simulink model "proxy_linux"  (R2017b)
settings: Solver=ode3  StartTime=0.0  StopTime=inf  FixedStep=0.01  RelTol=1e-3  EnableMultiTasking=on
model workspace (MAT data in the model file):
  SL_ROS_VariableLengthArrays_MaxSizes.CommonInfo.ArrayTruncateAction = 'EmitWarning'
  SL_ROS_VariableLengthArrays_MaxSizes.MsgTypeMap = containers.Map
  SL_ROS_VariableLengthArrays_MaxSizes.MsgTypeMap.serialization.keys = {'std_msgs/Float32MultiArray'}
  SL_ROS_VariableLengthArrays_MaxSizes.MsgTypeMap.serialization.values{1}.PropertyName = 'Data'
  SL_ROS_VariableLengthArrays_MaxSizes.MsgTypeMap.serialization.values{1}.DataType = 'single'
  SL_ROS_VariableLengthArrays_MaxSizes.MsgTypeMap.serialization.values{1}.MaxLength = 2
  SL_ROS_VariableLengthArrays_MaxSizes.MsgTypeMap.serialization.uniformity = 0
  SL_ROS_VariableLengthArrays_MaxSizes.MsgTypeMap.serialization.keyType = 'char'
  SL_ROS_VariableLengthArrays_MaxSizes.MsgTypeMap.serialization.valueType = 'any'
undefined symbols (not defined in the file or in its folder): ampliFactor, ampliFactorDistal, ampliFactorMiddle, filt
libraries: robotlib x11, simulink_extras x11, simulink x8, etargetslib x4, dspnetwork x4
(part 1 of 6)
settings Model: Creator=Centauro  LastModifiedBy=Centauro
settings DataIOCC: LimitDataPoints=on  SaveFormat=Array
settings OptimizationCC: PassReuseOutputArgsThreshold=0  MaxStackSize=64
settings DebuggingCC: ParameterTunabilityLossMsg=error  SFUnexpectedBacktrackingDiag=warning  SFNoUnconditionalDefaultTransitionDiag=warning  SFExecutionAtInitializationDiag=none
settings HardwareCC: ProdBitPerPointer=32  ProdBitPerSizeT=32  ProdBitPerPtrDiffT=32  ProdLargestAtomicFloat=None  ProdIntDivRoundTo=Undefined  ProdEndianess=Unspecified  ProdWordSize=32  ProdHWDeviceType=Generic->Unspecified (assume 32-bit Generic)  UseEmbeddedCoderFeatures=off
settings ModelReferenceCC: PropagateSignalLabelsOutOfModel=off
settings SFSimCC: MATLABDynamicMemAlloc=off
settings RTWCC: SystemTargetFile=ert.tlc  HardwareBoard=Robot Operating System (ROS)  TemplateMakefile=ert_default_tmf  GenerateReport=on  Toolchain=Catkin  LaunchReport=on  TargetLang=C++
settings CodeAppCC: ForceParamTrailComments=on  OperatorAnnotations=on
settings ERTTargetCC: ERTCustomFileBanners=off  SupportContinuousTime=on  SupportNonInlinedSFcns=on  RemoveResetFunc=off  ModelStepFunctionPrototypeControlCompliant=off
settings ConfigComp: CovMetricSettings=dw  CovHtmlReporting=on  CovSaveCumulativeToWorkspaceVar=on  CovSaveSingleToWorkspaceVar=on  CovExternalEMLEnable=off

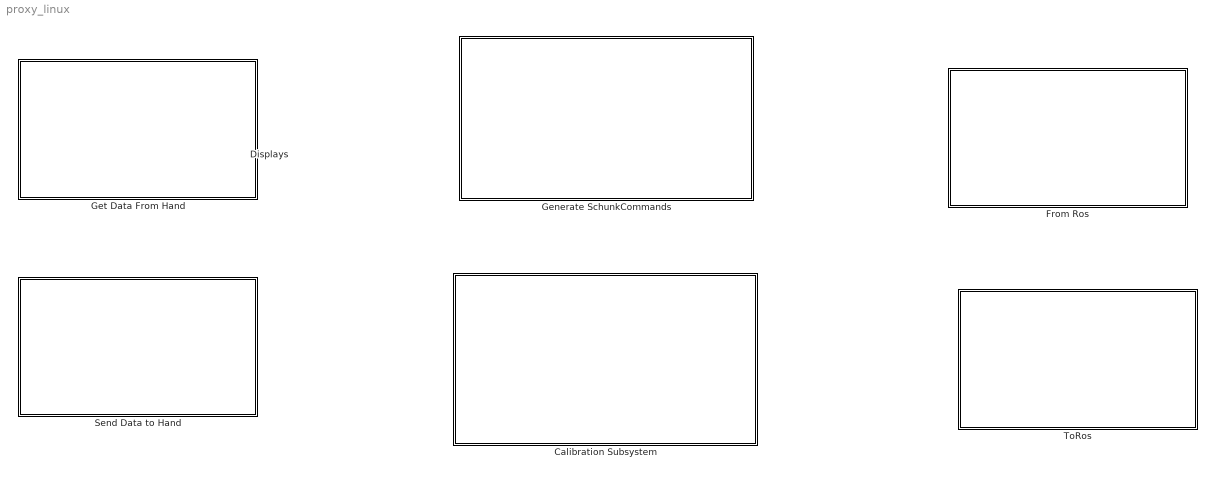
== system proxy_linux ==
  Calibration Subsystem : Subsystem
  "Displays " : Subsystem
  From Ros : Subsystem
  "Generate SchunkCommands " : Subsystem
  Get Data From Hand : Subsystem
  Send Data to Hand : Subsystem
  ToRos : Subsystem

== system proxy_linux/Calibration Subsystem ==
  Bus Selector : BusSelector  OutputSignals=Data
  Chart : Stateflow chart  Commented=on  TreatAsAtomicUnit=on
  Constant : Constant  Value=true  OutDataTypeStr=boolean
  Display : Display
  From1 : From  Commented=on  GotoTag=Index_Precalibration  TagVisibility=global
  From2 : From  Commented=on  GotoTag=Middle_Precalibration
  Goto1 : Goto  Commented=on  GotoTag=CalibrationSignal  TagVisibility=global
  Goto2 : Goto  Commented=on  GotoTag=IndexCalibrationOffset  TagVisibility=global
  Goto3 : Goto  Commented=on  GotoTag=MiddleCalibrationOffset  TagVisibility=global
  Logical Operator : Logic  Operator=NOT  AllPortsSameDT=off  OutDataTypeStr=boolean
  Manual Switch : ManualSwitch  CurrentSetting=0
  Memory : Memory  Commented=on
  Memory1 : Memory  Commented=on
  Memory2 : Memory  Commented=on
  Subscribe1 : robotlib/Subscribe  SourceLibraryInfo=This block requires Robotics System Toolbox  topicSource=Select from ROS network  topic=/left_hand/button_1  messageType=std_msgs/Bool  sampleTime=0.01  messageQueueLength=1
      settings: SourceProductBaseCode=RO
  Terminator : Terminator
  tag scope: CalibrationSignal=global
  wires:
  Subscribe1/1 -> Terminator/1
  Subscribe1/2 -> Bus Selector/1
  From1/1 -> Chart/1(IndexPrescaler)
  From2/1 -> Chart/2(MiddlePrescaler)
  Chart/2(MiddleOffset) -> Memory1/1
  Chart/1(IndexOffset) -> Memory/1
  Chart/3(CalibrationDone) -> Memory2/1
  Memory/1 -> Goto2/1
  Memory1/1 -> Goto3/1
  Memory2/1 -> Goto1/1
  Logical Operator/1 -> [CalibrationSignal], Chart/3(Calibration), Display/1
  Manual Switch/1 -> Logical Operator/1
  Bus Selector/1 -> Manual Switch/2  "<Data>"
  Constant/1 -> Manual Switch/1

== system proxy_linux/Displays  ==
  Display{,1..3} (4 alike) : Display
  wires:
  [Forces] -> Display1/1
  [RotativePot] -> Display3/1
  [Header] -> Display/1
  [MotorsPot] -> Display2/1

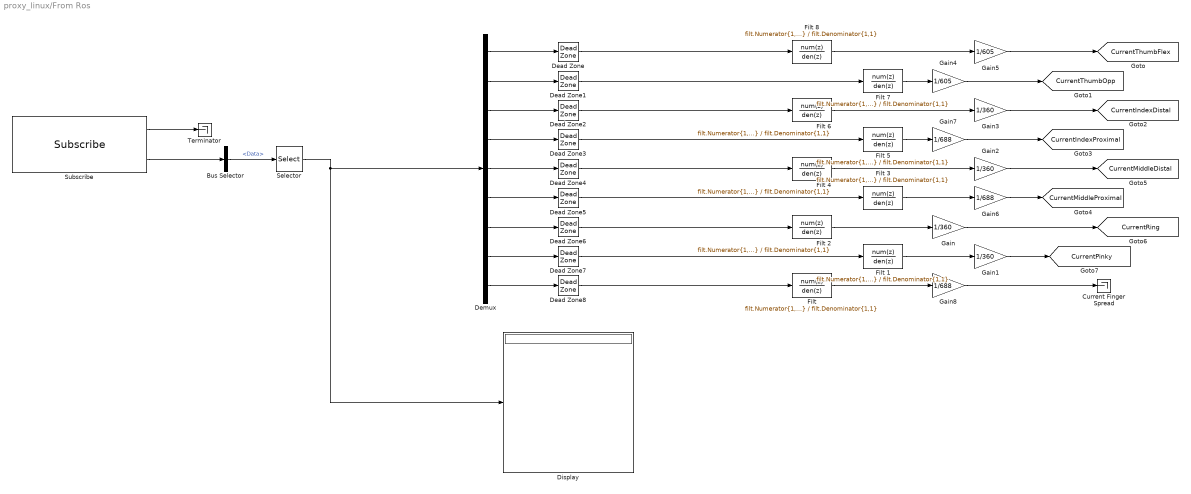
== system proxy_linux/From Ros ==
  Bus Selector : BusSelector  OutputSignals=Data
  Current Finger Spread : Terminator
  Dead Zone{,1..8} (9 alike) : DeadZone  LowerValue=-30  UpperValue=30  SaturateOnIntegerOverflow=on
  Demux : Demux  Outputs=9
  Display : Display
  Filt {,1..8} (9 alike) : DiscreteTransferFcn  Numerator=filt.Numerator{1,1}  Denominator=filt.Denominator{1,1}  SampleTime=0.01
  Gain{,1..3} (4 alike) : Gain  Gain=1/360
  Gain4 : Gain  Gain=1/605
  Gain5 : Gain  Gain=1/605
  Gain6 : Gain  Gain=1/688
  Gain7 : Gain  Gain=1/688
  Gain8 : Gain  Gain=1/688
  Selector : Selector  IndexOptions=Index vector (dialog)  Indices=[1 2 3 4 5 6 7 8 9]  OutputSizes=1
  Subscribe : robotlib/Subscribe  SourceLibraryInfo=This block requires Robotics System Toolbox  topicSource=Select from ROS network  topic=/svh_controller/channel_currents  messageType=std_msgs/Float64MultiArray  sampleTime=0.01  messageQueueLength=1
      settings: SourceProductBaseCode=RO
  Terminator : Terminator
  tag scope: CurrentIndexDistal=global, CurrentIndexProximal=global, CurrentMiddleDistal=global, CurrentMiddleProximal=global, CurrentPinky=global, CurrentRing=global, CurrentThumbFlex=global, CurrentThumbOpp=global
  wires:
  Subscribe/1 -> Terminator/1
  Subscribe/2 -> Bus Selector/1
  Bus Selector/1 -> Selector/1  "<Data>"
  Selector/1 -> Demux/1, Display/1
  Demux/1 -> Dead Zone/1
  Demux/2 -> Dead Zone1/1
  Demux/3 -> Dead Zone2/1
  Demux/4 -> Dead Zone3/1
  Demux/6 -> Dead Zone5/1
  Demux/5 -> Dead Zone4/1
  Demux/7 -> Dead Zone6/1
  Demux/8 -> Dead Zone7/1
  Demux/9 -> Dead Zone8/1
  "Filt "/1 -> Gain8/1
  Filt 1/1 -> Gain1/1
  Filt 2/1 -> Gain/1
  Filt 4/1 -> Gain2/1
  Filt 5/1 -> Gain7/1
  Filt 6/1 -> Gain3/1
  Filt 7/1 -> Gain4/1
  Filt 8/1 -> Gain5/1
  Gain1/1 -> [CurrentPinky]
  Gain/1 -> [CurrentRing]
  Filt 3/1 -> Gain6/1
  Gain2/1 -> [CurrentMiddleDistal]
  Gain3/1 -> [CurrentIndexDistal]
  Gain5/1 -> [CurrentThumbFlex]
  Gain4/1 -> [CurrentThumbOpp]
  Gain7/1 -> [CurrentIndexProximal]
  Gain6/1 -> [CurrentMiddleProximal]
  Gain8/1 -> Current Finger Spread/1
  Dead Zone/1 -> Filt 8/1
  Dead Zone1/1 -> Filt 7/1
  Dead Zone2/1 -> Filt 6/1
  Dead Zone3/1 -> Filt 5/1
  Dead Zone4/1 -> Filt 4/1
  Dead Zone5/1 -> Filt 3/1
  Dead Zone6/1 -> Filt 2/1
  Dead Zone7/1 -> Filt 1/1
  Dead Zone8/1 -> "Filt "/1

== system proxy_linux/Generate SchunkCommands  ==
  Finger Spread : Subsystem
  Index : Subsystem
  Index Finger : Subsystem  Commented=on
  Middle Finger : Subsystem
  Pinky : Subsystem
  "Ring " : Subsystem
  Thumb : Subsystem

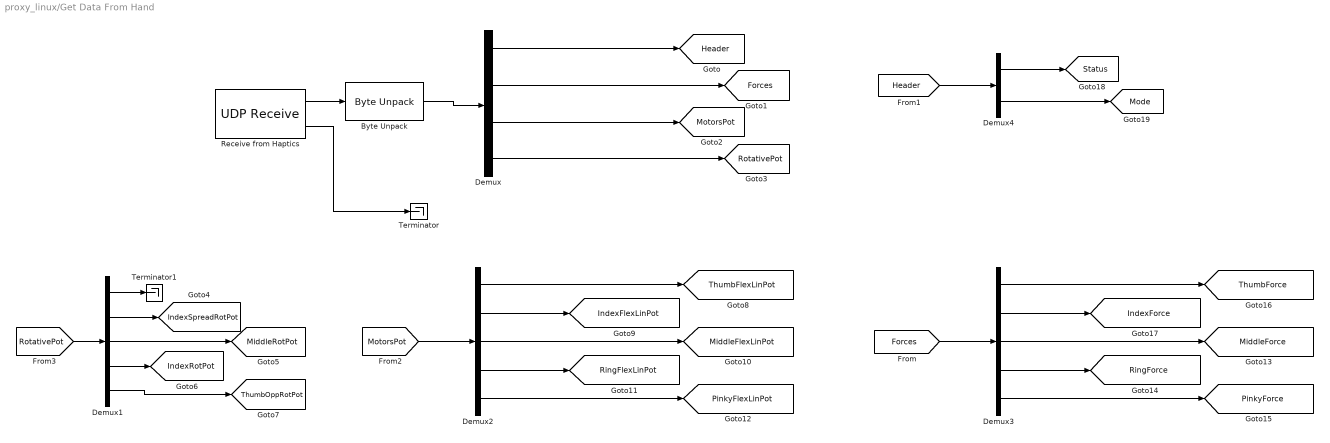
== system proxy_linux/Get Data From Hand ==
  Byte Unpack : etargetslib/Byte Unpack  dimensions={[17]}  datatypes={'single'}  byteAlign=1
  Demux : Demux  Outputs=[2, 5, 5, 5]
  Demux1 : Demux  Outputs=5
  Demux2 : Demux  Outputs=5
  Demux3 : Demux  Outputs=5
  Demux4 : Demux  Outputs=2
  Receive from Haptics : dspnetwork/UDP Receive  localURL='0.0.0.0'  localPort=15001  remoteURL=RightHandAddress  remotePort=-1  recvBufferSize=17*4  dims=17*4  signalDatatype=uint8  isVarSize=off  showBlockingTime=on  blockingTime=inf  sampletime=0.01  blockPlatform=HOST
      settings: SourceProductName=DSP System Toolbox  SourceProductBaseCode=DS
  Terminator : Terminator
  Terminator1 : Terminator
  tag scope: Forces=global, Header=global, IndexFlexLinPot=global, IndexForce=global, IndexRotPot=global, IndexSpreadRotPot=global, MiddleFlexLinPot=global, MiddleForce=global, MiddleRotPot=global, Mode=global, MotorsPot=global, PinkyFlexLinPot=global, PinkyForce=global, RingFlexLinPot=global, RingForce=global, RotativePot=global, Status=global, ThumbFlexLinPot=global, ThumbForce=global, ThumbOppRotPot=global
  wires:
  Demux/3 -> [MotorsPot]
  Demux/1 -> [Header]
  Demux/4 -> [RotativePot]
  Demux/2 -> [Forces]
  Receive from Haptics/2 -> Terminator/1
  [RotativePot] -> Demux1/1
  Demux1/2 -> [IndexSpreadRotPot]
  Demux1/3 -> [MiddleRotPot]
  Demux1/4 -> [IndexRotPot]
  Demux1/5 -> [ThumbOppRotPot]
  Demux1/1 -> Terminator1/1
  Demux2/1 -> [ThumbFlexLinPot]
  Demux2/2 -> [IndexFlexLinPot]
  [MotorsPot] -> Demux2/1
  Demux2/3 -> [MiddleFlexLinPot]
  Demux2/4 -> [RingFlexLinPot]
  Demux2/5 -> [PinkyFlexLinPot]
  Demux3/1 -> [ThumbForce]
  Demux3/2 -> [IndexForce]
  [Forces] -> Demux3/1
  Demux3/3 -> [MiddleForce]
  Demux3/4 -> [RingForce]
  Demux3/5 -> [PinkyForce]
  [Header] -> Demux4/1
  Demux4/1 -> [Status]
  Demux4/2 -> [Mode]
  Byte Unpack/1 -> Demux/1
  Receive from Haptics/1 -> Byte Unpack/1

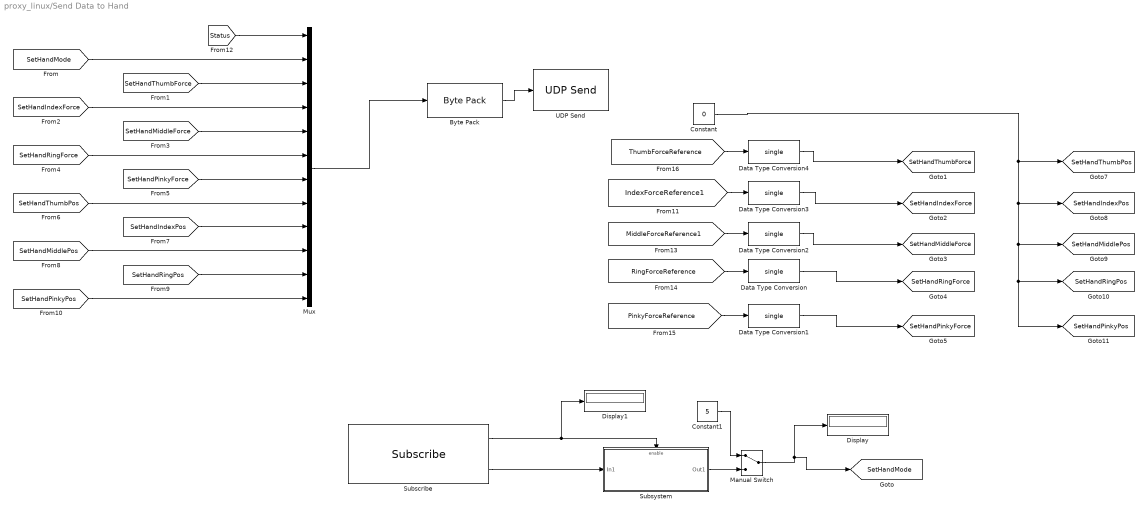
== system proxy_linux/Send Data to Hand ==
  Byte Pack : etargetslib/Byte Pack  datatypes={'single'}  byteAlign=1
  Constant : Constant  Value=0  OutDataTypeStr=single
  Constant1 : Constant  Value=5  OutDataTypeStr=single
  Data Type Conversion{,1..4} (5 alike) : DataTypeConversion  OutDataTypeStr=single
  Display : Display
  Display1 : Display
  Manual Switch : ManualSwitch
  Mux : Mux  Inputs=12
  Subscribe : robotlib/Subscribe  SourceLibraryInfo=This block requires Robotics System Toolbox  topicSource=Specify your own  topic=/manual_commands/rh_mode  messageType=std_msgs/Float64  sampleTime=-1  messageQueueLength=1
      settings: SourceProductBaseCode=RO
  Subsystem : Subsystem
  UDP Send : dspnetwork/UDP Send  remoteURL=RightHandAddress  remotePort=12000  localURL='0.0.0.0'  localPortSource=Automatically determine  localPort=-1  sampletime=-1  blockPlatform=HOST  separateLengthPort=0
      settings: SourceProductName=DSP System Toolbox  SourceProductBaseCode=DS
  tag scope: SetHandIndexForce=global, SetHandIndexPos=global, SetHandMiddleForce=global, SetHandMiddlePos=global, SetHandMode=global, SetHandPinkyForce=global, SetHandPinkyPos=global, SetHandRingForce=global, SetHandRingPos=global, SetHandThumbForce=global, SetHandThumbPos=global
  wires:
  Byte Pack/1 -> UDP Send/1
  [SetHandMode] -> Mux/2
  [SetHandThumbForce] -> Mux/3
  [SetHandIndexForce] -> Mux/4
  [SetHandRingForce] -> Mux/6
  [SetHandMiddleForce] -> Mux/5
  [SetHandPinkyForce] -> Mux/7
  [SetHandThumbPos] -> Mux/8
  [SetHandIndexPos] -> Mux/9
  [SetHandMiddlePos] -> Mux/10
  [SetHandRingPos] -> Mux/11
  [SetHandPinkyPos] -> Mux/12
  [Status] -> Mux/1
  [ThumbForceReference] -> Data Type Conversion4/1
  [RingForceReference] -> Data Type Conversion/1
  [PinkyForceReference] -> Data Type Conversion1/1
  [MiddleForceReference1] -> Data Type Conversion2/1
  [IndexForceReference1] -> Data Type Conversion3/1
  Constant/1 -> [SetHandThumbPos], [SetHandIndexPos], [SetHandMiddlePos], [SetHandRingPos], [SetHandPinkyPos]
  Mux/1 -> Byte Pack/1
  Subscribe/2 -> Subsystem/1(In1)
  Subscribe/1 -> Display1/1, Subsystem/Enable
  Data Type Conversion/1 -> [SetHandRingForce]
  Data Type Conversion1/1 -> [SetHandPinkyForce]
  Data Type Conversion2/1 -> [SetHandMiddleForce]
  Data Type Conversion3/1 -> [SetHandIndexForce]
  Data Type Conversion4/1 -> [SetHandThumbForce]
  Subsystem/1(Out1) -> Manual Switch/2
  Constant1/1 -> Manual Switch/1
  Manual Switch/1 -> [SetHandMode], Display/1

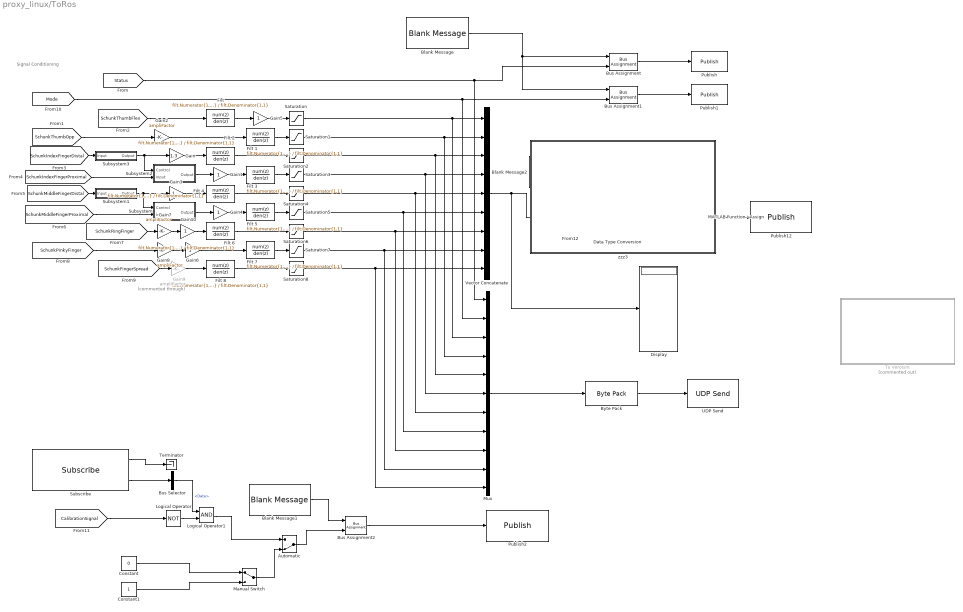
== system proxy_linux/ToRos ==
  note: Signal Conditioning
  "Automatic " : ManualSwitch  CurrentSetting=0
  Blank Message : robotlib/Blank Message  SourceLibraryInfo=This block requires Robotics System Toolbox  messageType=std_msgs/Float32  SampleTime=0.01
      settings: SourceProductBaseCode=RO
  Blank Message1 : robotlib/Blank Message  SourceLibraryInfo=This block requires Robotics System Toolbox  messageType=std_msgs/Bool  SampleTime=inf
      settings: SourceProductBaseCode=RO
  Blank Message2 : robotlib/Blank Message  SourceLibraryInfo=This block requires Robotics System Toolbox  messageType=sensor_msgs/JointState  SampleTime=inf
      settings: SourceProductBaseCode=RO
  Bus Assignment : BusAssignment  AssignedSignals=Data
  Bus Assignment1 : BusAssignment  AssignedSignals=Data
  Bus Assignment2 : BusAssignment  AssignedSignals=Data
  Bus Selector : BusSelector  OutputSignals=Data
  Byte Pack : etargetslib/Byte Pack  datatypes={'single'}  byteAlign=1
  Constant : Constant  Value=0  OutDataTypeStr=boolean
  Constant1 : Constant  OutDataTypeStr=boolean
  Data Type Conversion : DataTypeConversion  OutDataTypeStr=uint32
  Display : Display
  Filt {,1..8} (9 alike) : DiscreteTransferFcn  Numerator=filt.Numerator{1,1}  Denominator=filt.Denominator{1,1}  SampleTime=0.01
  Gain : Gain  Gain=1.3
  Gain{1,3..6,10} (6 alike) : Gain
  Gain2 : Gain  Gain=ampliFactor
  Gain7 : Gain  Gain=ampliFactor
  Gain8 : Gain  Gain=ampliFactor
  Gain9 : Gain  Commented=through  Gain=ampliFactor
  Logical Operator : Logic  Operator=NOT  AllPortsSameDT=off  OutDataTypeStr=boolean
  Logical Operator1 : Logic  AllPortsSameDT=off  OutDataTypeStr=boolean
  MATLAB Function - Assign : MATLAB Function  TreatAsAtomicUnit=on
  Manual Switch : ManualSwitch
  Mux : Mux  Inputs=11
  Publish : robotlib/Publish  SourceLibraryInfo=This block requires Robotics System Toolbox  topicSource=Specify your own  topic=/MatlabStatus  messageType=std_msgs/Float32  messageQueueLength=1
      settings: SourceProductBaseCode=RO
  Publish1 : robotlib/Publish  SourceLibraryInfo=This block requires Robotics System Toolbox  topicSource=Specify your own  topic=/MatlabMode  messageType=std_msgs/Float32  messageQueueLength=1
      settings: SourceProductBaseCode=RO
  Publish12 : robotlib/Publish  SourceLibraryInfo=This block requires Robotics System Toolbox  topicSource=Specify your own  topic=/scan  messageType=sensor_msgs/JointState  messageQueueLength=1
      settings: SourceProductBaseCode=RO
  Publish2 : robotlib/Publish  SourceLibraryInfo=This block requires Robotics System Toolbox  topicSource=Specify your own  topic=/trigger_exo_hand  messageType=std_msgs/Bool  messageQueueLength=1
      settings: SourceProductBaseCode=RO
  Saturation : Saturate  UpperLimit=0.97  LowerLimit=0
  Saturation1 : Saturate  UpperLimit=0.99  LowerLimit=0
  Saturation2 : Saturate  UpperLimit=1.33  LowerLimit=0
  Saturation3 : Saturate  UpperLimit=0.80  LowerLimit=0
  Saturation4 : Saturate  UpperLimit=1.33  LowerLimit=0
  Saturation5 : Saturate  UpperLimit=0.80  LowerLimit=0
  Saturation6 : Saturate  UpperLimit=0.98  LowerLimit=0
  Saturation7 : Saturate  UpperLimit=0.98  LowerLimit=0
  Saturation8 : Saturate  UpperLimit=0.30  LowerLimit=0.05
  Subscribe : robotlib/Subscribe  SourceLibraryInfo=This block requires Robotics System Toolbox  topicSource=Specify your own  topic=/manual_commands/start  messageType=std_msgs/Bool  sampleTime=0.01  messageQueueLength=1
      settings: SourceProductBaseCode=RO
  Subsystem : Subsystem
  Subsystem1 : Subsystem
  Subsystem2 : Subsystem
  Subsystem3 : Subsystem
  Terminator : Terminator
  To Verosim : Subsystem  Commented=on
  UDP Send : dspnetwork/UDP Send  remoteURL=Verosim  remotePort=15000  localURL='0.0.0.0'  localPortSource=Automatically determine  localPort=-1  sampletime=-1  blockPlatform=HOST  separateLengthPort=0
      settings: SourceProductName=DSP System Toolbox  SourceProductBaseCode=DS
  Vector Concatenate : Concatenate  NumInputs=9
  zzz3 : Subsystem  TreatAsAtomicUnit=on
      settings: OpenFcn=% no-op
      mask Display: disp('')
  wires:
  Bus Assignment/1 -> Publish/1
  Blank Message/1 -> Bus Assignment1/1, Bus Assignment/1
  Bus Assignment1/1 -> Publish1/1
  MATLAB Function - Assign/1(msg) -> Publish12/1
  "Filt "/1 -> Gain5/1
  Filt 5/1 -> Saturation5/1
  Filt 6/1 -> Saturation6/1
  Filt 3/1 -> Saturation3/1
  Filt 2/1 -> Saturation2/1
  Filt 4/1 -> Saturation4/1
  Filt 8/1 -> Saturation8/1
  Filt 1/1 -> Saturation1/1
  Filt 7/1 -> Saturation7/1
  [SchunkThumbFlex] -> "Filt "/1
  Gain7/1 -> Gain10/1
  [SchunkFingerSpread] -> Gain9/1
  Gain2/1 -> Filt 1/1
  [SchunkPinkyFinger] -> Gain8/1
  [SchunkThumbOpp] -> Gain2/1
  [SchunkRingFinger] -> Gain7/1
  Gain8/1 -> Gain6/1
  Gain9/1 -> Filt 8/1
  Subsystem3/1(Output) -> Subsystem2/1(Control), Gain/1
  [SchunkMiddleFingerProximal] -> Subsystem/2(Input)
  Bus Assignment2/1 -> Publish2/1
  [CalibrationSignal] -> Logical Operator/1
  Manual Switch/1 -> "Automatic "/2
  Blank Message1/1 -> Bus Assignment2/1
  Constant/1 -> Manual Switch/1
  "Automatic "/1 -> Bus Assignment2/2
  Constant1/1 -> Manual Switch/2
  Vector Concatenate/1 -> Display/1, MATLAB Function - Assign/2(u)
  Subsystem/1("Output ") -> Gain4/1
  [SchunkMiddleFingerDistal] -> Subsystem1/1(Input)
  Subsystem1/1(Output) -> Subsystem/1(Control), Gain3/1
  Saturation/1 -> Mux/3, Vector Concatenate/1
  Saturation1/1 -> Mux/4, Vector Concatenate/2
  Byte Pack/1 -> UDP Send/1
  [Mode] -> Bus Assignment1/2, Mux/2
  [Status] -> Bus Assignment/2, Mux/1
  Saturation5/1 -> Mux/8, Vector Concatenate/6
  Saturation8/1 -> Mux/11, Vector Concatenate/9
  Saturation2/1 -> Mux/5, Vector Concatenate/3
  Saturation3/1 -> Mux/6, Vector Concatenate/4
  Saturation6/1 -> Mux/9, Vector Concatenate/7
  Saturation7/1 -> Mux/10, Vector Concatenate/8
  Saturation4/1 -> Mux/7, Vector Concatenate/5
  Mux/1 -> Byte Pack/1
  Subsystem2/1("Output ") -> Gain1/1
  [SchunkIndexFingerProximal] -> Subsystem2/2(Input)
  [SchunkIndexFingerDistal] -> Subsystem3/1(Input)
  Logical Operator/1 -> Logical Operator1/2
  Logical Operator1/1 -> "Automatic "/1
  Bus Selector/1 -> Logical Operator1/1  "<Data>"
  Subscribe/1 -> Terminator/1
  Subscribe/2 -> Bus Selector/1
  Gain/1 -> Filt 2/1
  Blank Message2/1 -> MATLAB Function - Assign/1(blankMessage)
  Data Type Conversion/1 -> MATLAB Function - Assign/3(timeStamp)
  [Status] -> Data Type Conversion/1
  Gain1/1 -> Filt 3/1
  Gain3/1 -> Filt 4/1
  Gain4/1 -> Filt 5/1
  Gain5/1 -> Saturation/1
  Gain6/1 -> Filt 7/1
  Gain10/1 -> Filt 6/1

== system proxy_linux/Generate SchunkCommands /Finger Spread ==
  Constant : Constant  Value=0.30  OutDataTypeStr=single
  Constant1 : Constant  Value=0.10  OutDataTypeStr=single
  Display : Display
  MATLAB Function : MATLAB Function  TreatAsAtomicUnit=on
  Manual Switch : ManualSwitch
  Mux : Mux  Inputs=2
  Sum : Sum  Inputs=|++
  calibration1 : Subsystem
  tag scope: SchunkFingerSpread=global
  wires:
  [IndexSpreadRotPot] -> calibration1/1(In1), MATLAB Function/1(u)
  Constant/1 -> Manual Switch/2
  MATLAB Function/1(y) -> Manual Switch/1
  calibration1/1(Out1) -> Mux/2, MATLAB Function/2(calib)
  Mux/1 -> Display/1
  Manual Switch/1 -> Sum/1
  Sum/1 -> Mux/1, [SchunkFingerSpread]
  Constant1/1 -> Sum/2

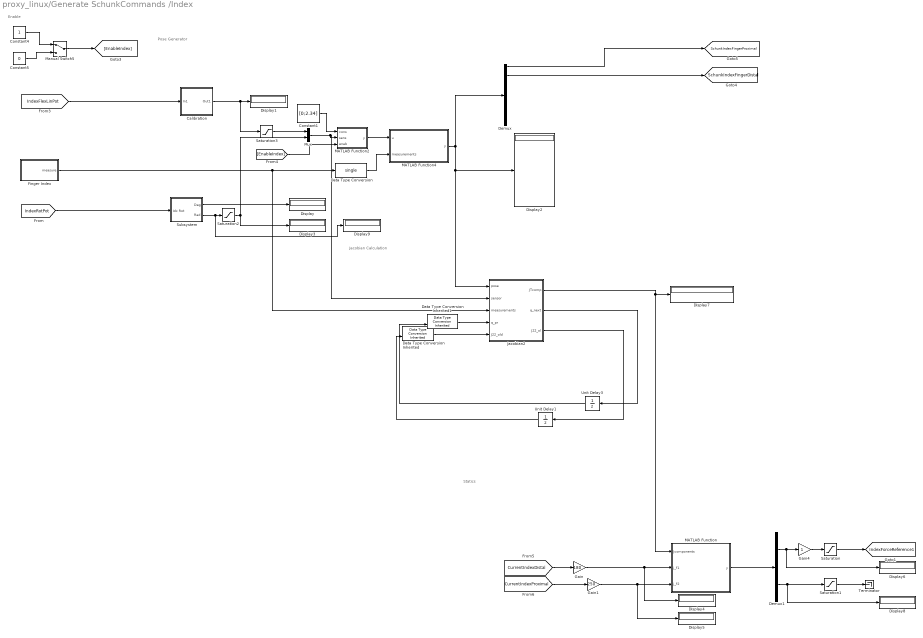
== system proxy_linux/Generate SchunkCommands /Index ==
  note: Enable
  note: Statics
  note: Jacobian Calculation
  note: Pose Generator
  Calibration : Subsystem
  Constant1 : Constant  Value=[0;2.34]  OutDataTypeStr=single
  Constant4 : Constant  OutDataTypeStr=single
  Constant5 : Constant  Value=0  OutDataTypeStr=single
  Data Type Conversion Inherited : simulink/Signal Attributes/Data Type Conversion Inherited  ConvertRealWorld=Real World Value  DoSatur=off
      settings: SourceProductName=Simulink  SourceProductBaseCode=SL
  Data Type Conversion Inherited1 : simulink/Signal Attributes/Data Type Conversion Inherited  ConvertRealWorld=Real World Value  DoSatur=off
      settings: SourceProductName=Simulink  SourceProductBaseCode=SL
  Data Type Conversion : DataTypeConversion  OutDataTypeStr=single
  Demux : Demux  Outputs=8
  Demux1 : Demux  Outputs=2
  Display{,1..9} (10 alike) : Display
  "Finger Index " : Subsystem
  Gain : Gain  Gain=180
  Gain1 : Gain  Gain=250
  Gain4 : Gain
  Jacobian2 : MATLAB Function  TreatAsAtomicUnit=on  SystemSampleTime=0.01
  MATLAB Function : MATLAB Function  TreatAsAtomicUnit=on
  MATLAB Function2 : MATLAB Function  TreatAsAtomicUnit=on
  MATLAB Function4 : MATLAB Function  TreatAsAtomicUnit=on
  Manual Switch5 : ManualSwitch
  Mux : Mux  Inputs=2
  Saturation : Saturate  UpperLimit=6  LowerLimit=-6
  Saturation1 : Saturate  UpperLimit=5  LowerLimit=-5
  Saturation2 : Saturate  UpperLimit=2.34  LowerLimit=-100
  Saturation3 : Saturate  UpperLimit=100  LowerLimit=0
  Subsystem : Subsystem
  Terminator : Terminator
  Unit Delay1 : UnitDelay  InitialCondition=-1  SampleTime=0.01
  Unit Delay3 : UnitDelay  InitialCondition=[0;2.3]  SampleTime=0.01
  tag scope: IndexForceReference1=global, SchunkIndexFingerDistal=global, SchunkIndexFingerProximal=global
  wires:
  Demux/1 -> [SchunkIndexFingerProximal]
  Demux/2 -> [SchunkIndexFingerDistal]
  [IndexRotPot] -> Subsystem/1(Idx Rot)
  Subsystem/1(Deg) -> Display/1
  Constant1/1 -> MATLAB Function2/1(cons)
  Subsystem/2(Rad) -> Display9/1, Saturation2/1
  Data Type Conversion/1 -> MATLAB Function4/2(measurements)
  MATLAB Function2/1(y) -> MATLAB Function4/1(u)
  Unit Delay3/1 -> Data Type Conversion Inherited1/2
  Jacobian2/3(J22_ol) -> Unit Delay1/1
  Data Type Conversion Inherited/1 -> Jacobian2/5(J22_old)
  Mux/1 -> Jacobian2/2(sensor), MATLAB Function2/2(sens)
  Unit Delay1/1 -> Data Type Conversion Inherited/2
  "Finger Index "/1(measure) -> Jacobian2/3(measurements), Data Type Conversion/1
  Data Type Conversion Inherited1/1 -> Jacobian2/4(q_pr)
  Jacobian2/2(q_next) -> Unit Delay3/1
  MATLAB Function4/1(y) -> Jacobian2/1(pose), Display2/1, Demux/1
  [CurrentIndexProximal] -> Gain1/1
  Gain/1 -> Display4/1, MATLAB Function/2(j_f1)
  [CurrentIndexDistal] -> Gain/1
  Saturation1/1 -> Terminator/1
  Demux1/2 -> Display8/1, Saturation1/1
  Gain1/1 -> Display5/1, MATLAB Function/3(j_f2)
  Demux1/1 -> Display6/1, Gain4/1
  Jacobian2/1(JTcomp) -> MATLAB Function/1(Jcomponents), Display7/1
  MATLAB Function/1(y) -> Demux1/1
  Saturation/1 -> [IndexForceReference1]
  Manual Switch5/1 -> [EnableIndex]
  Constant5/1 -> Manual Switch5/2
  Constant4/1 -> Manual Switch5/1
  [EnableIndex] -> MATLAB Function2/3(enab)
  Gain4/1 -> Saturation/1
  Saturation2/1 -> Mux/2, Display3/1
  Calibration/1(Out1) -> Saturation3/1, Display1/1
  [IndexFlexLinPot] -> Calibration/1(In1)
  Saturation3/1 -> Mux/1

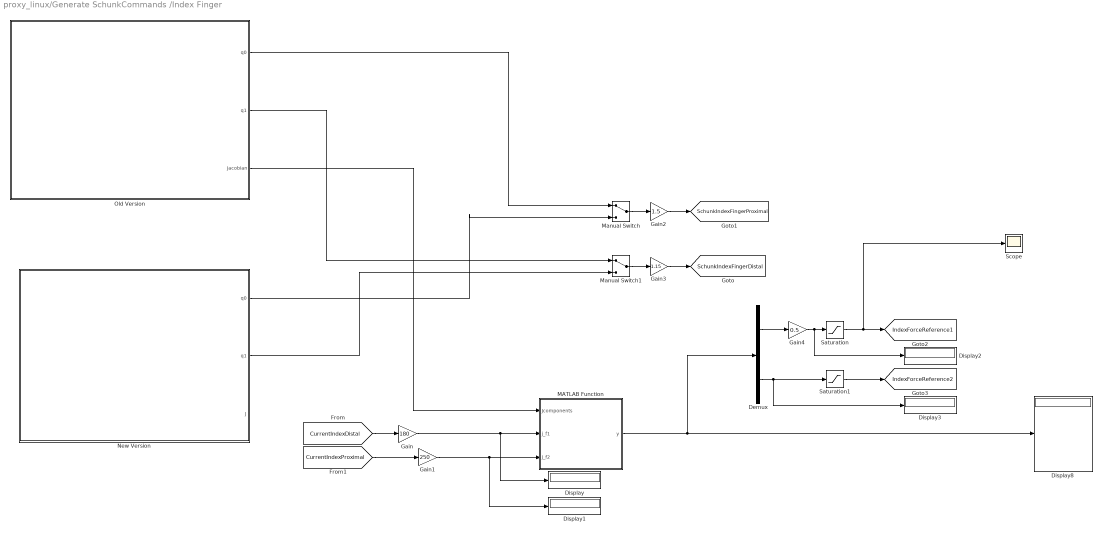
== system proxy_linux/Generate SchunkCommands /Index Finger ==
  Demux : Demux  Outputs=2
  Display{,1..3,8} (5 alike) : Display
  Gain : Gain  Gain=180
  Gain1 : Gain  Gain=250
  Gain2 : Gain  Gain=1.5
  Gain3 : Gain  Gain=1.15
  Gain4 : Gain  Gain=0.5
  MATLAB Function : MATLAB Function  TreatAsAtomicUnit=on
  Manual Switch : ManualSwitch
  Manual Switch1 : ManualSwitch
  New Version : Subsystem
  Old Version : Subsystem
  Saturation : Saturate  UpperLimit=5  LowerLimit=-5
  Saturation1 : Saturate  UpperLimit=5  LowerLimit=-5
  Scope : Scope
  tag scope: IndexForceReference1=global, IndexForceReference2=global, SchunkIndexFingerDistal=global, SchunkIndexFingerProximal=global
  wires:
  MATLAB Function/1(y) -> Demux/1, Display8/1
  Manual Switch1/1 -> Gain3/1
  Old Version/2(q1) -> Manual Switch1/1
  Manual Switch/1 -> Gain2/1
  Old Version/1(q0) -> Manual Switch/1
  New Version/1(q0) -> Manual Switch/2
  New Version/2(q1) -> Manual Switch1/2
  Demux/1 -> Gain4/1
  Demux/2 -> Display3/1, Saturation1/1
  [CurrentIndexDistal] -> Gain/1
  [CurrentIndexProximal] -> Gain1/1
  Saturation1/1 -> [IndexForceReference2]
  Saturation/1 -> Scope/1, [IndexForceReference1]
  Gain1/1 -> Display1/1, MATLAB Function/3(j_f2)
  Gain/1 -> Display/1, MATLAB Function/2(j_f1)
  Gain3/1 -> [SchunkIndexFingerDistal]
  Gain2/1 -> [SchunkIndexFingerProximal]
  Old Version/3(Jacobian) -> MATLAB Function/1(Jcomponents)
  Gain4/1 -> Display2/1, Saturation/1

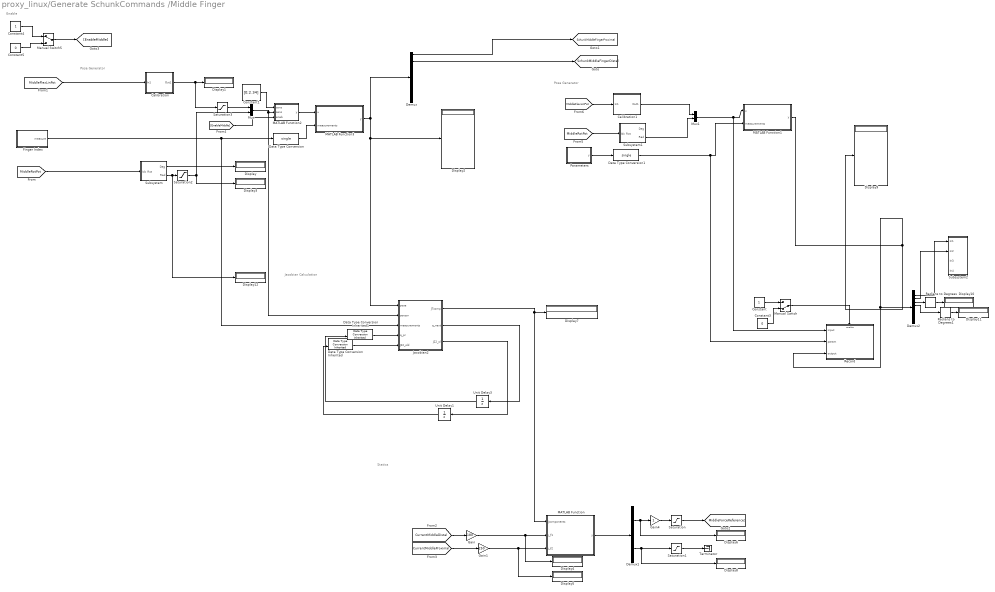
== system proxy_linux/Generate SchunkCommands /Middle Finger ==
  note: Enable
  note: Statics
  note: Jacobian Calculation
  note: Pose Generator
  note: Pose Generator
  Calibration : Subsystem
  Calibration1 : Subsystem
  Constant : Constant
  Constant1 : Constant  Value=[0;2.34]  OutDataTypeStr=single
  Constant3 : Constant  Value=0
  Constant4 : Constant  OutDataTypeStr=single
  Constant5 : Constant  Value=0  OutDataTypeStr=single
  Data Type Conversion Inherited : simulink/Signal Attributes/Data Type Conversion Inherited  ConvertRealWorld=Real World Value  DoSatur=off
      settings: SourceProductName=Simulink  SourceProductBaseCode=SL
  Data Type Conversion Inherited1 : simulink/Signal Attributes/Data Type Conversion Inherited  ConvertRealWorld=Real World Value  DoSatur=off
      settings: SourceProductName=Simulink  SourceProductBaseCode=SL
  Data Type Conversion : DataTypeConversion  OutDataTypeStr=single
  Data Type Conversion1 : DataTypeConversion  OutDataTypeStr=single
  Demux : Demux  Outputs=8
  Demux1 : Demux  Outputs=2
  Demux2 : Demux  Outputs=8
  Display{,1..12} (13 alike) : Display
  "Finger Index " : Subsystem
  Gain : Gain  Gain=180
  Gain1 : Gain  Gain=250
  Gain4 : Gain
  Jacobian2 : MATLAB Function  TreatAsAtomicUnit=on  SystemSampleTime=0.01
  MATLAB Function : MATLAB Function  TreatAsAtomicUnit=on
  MATLAB Function1 : MATLAB Function  TreatAsAtomicUnit=on
  MATLAB Function2 : MATLAB Function  TreatAsAtomicUnit=on
  MATLAB Function3 : MATLAB Function  TreatAsAtomicUnit=on
  Manual Switch : ManualSwitch  CurrentSetting=0
  Manual Switch5 : ManualSwitch
  Mux : Mux  Inputs=2
  Mux1 : Mux  Inputs=2
  Parameters : MATLAB Function  TreatAsAtomicUnit=on
  Radians to Degrees : simulink_extras/Transformations/Radians to Degrees
  Radians to Degrees1 : simulink_extras/Transformations/Radians to Degrees
  Record : Subsystem
  Saturation : Saturate  UpperLimit=6  LowerLimit=-6
  Saturation1 : Saturate  UpperLimit=5  LowerLimit=-5
  Saturation2 : Saturate  UpperLimit=2.34  LowerLimit=-100
  Saturation3 : Saturate  UpperLimit=100  LowerLimit=0
  Subsystem : Subsystem
  Subsystem1 : Subsystem
  Subsystem2 : Subsystem
  Terminator : Terminator
  Unit Delay1 : UnitDelay  InitialCondition=-1  SampleTime=0.01
  Unit Delay3 : UnitDelay  InitialCondition=[0;2.3]  SampleTime=0.01
  tag scope: MiddleForceReference1=global, SchunkMiddleFingerDistal=global, SchunkMiddleFingerProximal=global
  wires:
  Demux/1 -> [SchunkMiddleFingerProximal]
  Demux/2 -> [SchunkMiddleFingerDistal]
  [MiddleRotPot] -> Subsystem/1(Idx Rot)
  Subsystem/1(Deg) -> Display/1
  Constant1/1 -> MATLAB Function2/1(cons)
  Data Type Conversion/1 -> MATLAB Function3/2(measurements)
  MATLAB Function2/1(y) -> MATLAB Function3/1(u)
  Unit Delay3/1 -> Data Type Conversion Inherited1/2
  Jacobian2/3(J22_ol) -> Unit Delay1/1
  Data Type Conversion Inherited/1 -> Jacobian2/5(J22_old)
  Mux/1 -> Jacobian2/2(sensor), MATLAB Function2/2(sens)
  Unit Delay1/1 -> Data Type Conversion Inherited/2
  "Finger Index "/1(measure) -> Jacobian2/3(measurements), Data Type Conversion/1
  Data Type Conversion Inherited1/1 -> Jacobian2/4(q_pr)
  Jacobian2/2(q_next) -> Unit Delay3/1
  MATLAB Function3/1(y) -> Jacobian2/1(pose), Display2/1, Demux/1
  [CurrentMiddleProximal] -> Gain1/1
  Gain/1 -> Display4/1, MATLAB Function/2(j_f1)
  [CurrentMiddleDistal] -> Gain/1
  Saturation1/1 -> Terminator/1
  Demux1/2 -> Display8/1, Saturation1/1
  Gain1/1 -> Display5/1, MATLAB Function/3(j_f2)
  Demux1/1 -> Display6/1, Gain4/1
  Jacobian2/1(JTcomp) -> MATLAB Function/1(Jcomponents), Display7/1
  MATLAB Function/1(y) -> Demux1/1
  Saturation/1 -> [MiddleForceReference1]
  Manual Switch5/1 -> [EnableMiddle]
  Constant5/1 -> Manual Switch5/2
  Constant4/1 -> Manual Switch5/1
  [EnableMiddle] -> MATLAB Function2/3(enab)
  Gain4/1 -> Saturation/1
  Saturation2/1 -> Mux/2, Display3/1
  Calibration/1(Out1) -> Display1/1, Saturation3/1
  [MiddleFlexLinPot] -> Calibration/1(In1)
  Saturation3/1 -> Mux/1
  MATLAB Function1/1(y) -> Record/3(output), Demux2/1, Display9/1
  Demux2/3 -> Radians to Degrees/1
  Radians to Degrees/1 -> Display10/1
  Radians to Degrees1/1 -> Display11/1
  Demux2/4 -> Radians to Degrees1/1
  Subsystem/2(Rad) -> Display12/1, Saturation2/1
  [MiddleRotPot] -> Subsystem1/1(Idx Rot)
  Subsystem1/2(Rad) -> Mux1/2
  [MiddleFlexLinPot] -> Calibration1/1(In1)
  Calibration1/1(Out1) -> Mux1/1
  Parameters/1(y) -> Data Type Conversion1/1
  Demux2/1 -> Subsystem2/1(In1)
  Demux2/2 -> Subsystem2/2(In2)
  Manual Switch/1 -> Record/Enable
  Constant/1 -> Manual Switch/1
  Constant3/1 -> Manual Switch/2
  Data Type Conversion1/1 -> Record/2(param), MATLAB Function1/2(measurements)
  Mux1/1 -> Record/1(input), MATLAB Function1/1(u)

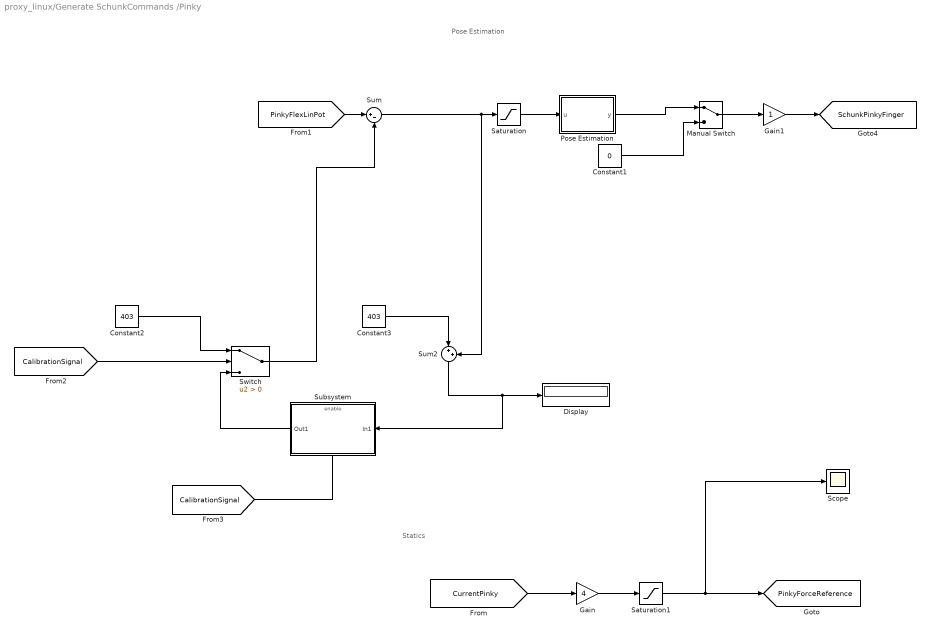
== system proxy_linux/Generate SchunkCommands /Pinky ==
  note: Pose Estimation
  note: Statics
  Constant1 : Constant  Value=0  OutDataTypeStr=single
  Constant2 : Constant  Value=403  OutDataTypeStr=single
  Constant3 : Constant  Value=403  OutDataTypeStr=single
  Display : Display
  Gain : Gain  Gain=4
  Gain1 : Gain
  Manual Switch : ManualSwitch
  Pose Estimation : MATLAB Function  TreatAsAtomicUnit=on
  Saturation : Saturate  UpperLimit=950  LowerLimit=0
  Saturation1 : Saturate  UpperLimit=5  LowerLimit=-5
  Scope : Scope
  Subsystem : Subsystem
  Sum : Sum  Inputs=|+-
  Sum2 : Sum  Inputs=|++
  Switch : Switch  Criteria=u2 > Threshold
  tag scope: PinkyForceReference=global, SchunkPinkyFinger=global
  wires:
  Saturation/1 -> Pose Estimation/1(u)
  Manual Switch/1 -> Gain1/1
  Pose Estimation/1(y) -> Manual Switch/1
  Constant1/1 -> Manual Switch/2
  Gain/1 -> Saturation1/1
  [CurrentPinky] -> Gain/1
  Saturation1/1 -> Scope/1, [PinkyForceReference]
  Constant2/1 -> Switch/1
  Subsystem/1(Out1) -> Switch/3
  Constant3/1 -> Sum2/1
  [CalibrationSignal] -> Subsystem/Enable
  Switch/1 -> Sum/2
  Sum2/1 -> Display/1, Subsystem/1(In1)
  [CalibrationSignal] -> Switch/2
  Sum/1 -> Sum2/2, Saturation/1
  [PinkyFlexLinPot] -> Sum/1
  Gain1/1 -> [SchunkPinkyFinger]

== system proxy_linux/Generate SchunkCommands /Ring  ==
  note: Statics
  note: Pose Estimation
  Constant1 : Constant  Value=0  OutDataTypeStr=single
  Gain : Gain  Gain=6
  Manual Switch : ManualSwitch
  Pose Estimation : MATLAB Function  TreatAsAtomicUnit=on
  Saturation : Saturate  UpperLimit=950  LowerLimit=0
  Saturation1 : Saturate  UpperLimit=5  LowerLimit=-5
  Sum : Sum  Inputs=|+-
  calibration : Subsystem
  tag scope: RingForceReference=global, SchunkRingFinger=global
  wires:
  Constant1/1 -> Manual Switch/2
  Manual Switch/1 -> [SchunkRingFinger]
  Pose Estimation/1(y) -> Manual Switch/1
  Gain/1 -> Saturation1/1
  [CurrentRing] -> Gain/1
  Saturation1/1 -> [RingForceReference]
  Saturation/1 -> Pose Estimation/1(u)
  [RingFlexLinPot] -> Sum/1
  Sum/1 -> calibration/1(In1), Saturation/1
  calibration/1(Out1) -> Sum/2

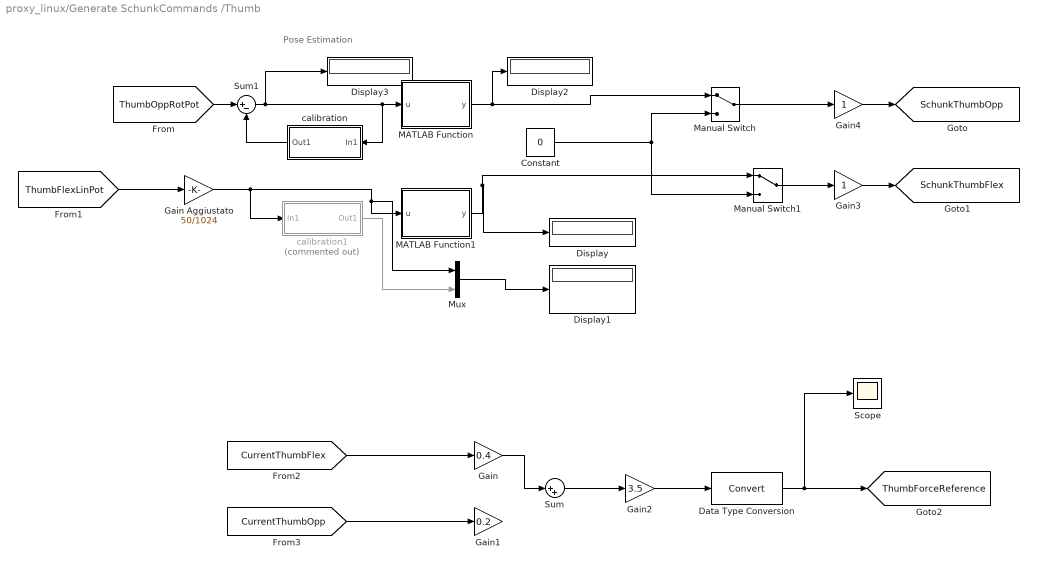
== system proxy_linux/Generate SchunkCommands /Thumb ==
  note: Pose Estimation
  Constant : Constant  Value=0  OutDataTypeStr=single
  Data Type Conversion : DataTypeConversion
  Display{,1..3} (4 alike) : Display
  Gain : Gain  Gain=0.4
  Gain Aggiustato : Gain  Gain=50/1024
  Gain1 : Gain  Gain=0.2
  Gain2 : Gain  Gain=3.5
  Gain3 : Gain
  Gain4 : Gain
  MATLAB Function : MATLAB Function  TreatAsAtomicUnit=on
  MATLAB Function1 : MATLAB Function  TreatAsAtomicUnit=on
  Manual Switch : ManualSwitch
  Manual Switch1 : ManualSwitch
  Mux : Mux  Inputs=2
  Scope : Scope
  Sum : Sum  Inputs=|++
  Sum1 : Sum  Inputs=|+-
  calibration : Subsystem
  calibration1 : Subsystem  Commented=on
  tag scope: SchunkThumbFlex=global, SchunkThumbOpp=global, ThumbForceReference=global
  wires:
  MATLAB Function1/1(y) -> Manual Switch1/1, Display/1
  Manual Switch/1 -> Gain4/1
  MATLAB Function/1(y) -> Display2/1, Manual Switch/1
  Manual Switch1/1 -> Gain3/1
  Constant/1 -> Manual Switch1/2, Manual Switch/2
  [CurrentThumbFlex] -> Gain/1
  [CurrentThumbOpp] -> Gain1/1
  Gain/1 -> Sum/1
  Sum/1 -> Gain2/1
  Gain2/1 -> Data Type Conversion/1
  Data Type Conversion/1 -> Scope/1, [ThumbForceReference]
  Gain3/1 -> [SchunkThumbFlex]
  Gain4/1 -> [SchunkThumbOpp]
  calibration/1(Out1) -> Sum1/2
  [ThumbOppRotPot] -> Sum1/1
  Sum1/1 -> Display3/1, calibration/1(In1), MATLAB Function/1(u)
  [ThumbFlexLinPot] -> Gain Aggiustato/1
  calibration1/1(Out1) -> Mux/2
  Mux/1 -> Display1/1
  Gain Aggiustato/1 -> calibration1/1(In1), Mux/1, MATLAB Function1/1(u)

== system proxy_linux/Send Data to Hand/Subsystem ==
  In1 : Inport
  Enable : EnablePort
  Bus Selector : BusSelector  OutputSignals=Data
  Data Type Conversion : DataTypeConversion  OutDataTypeStr=single
  Out1 : Outport
  wires:
  In1/1 -> Bus Selector/1
  Data Type Conversion/1 -> Out1/1
  Bus Selector/1 -> Data Type Conversion/1  "<Data>"

== system proxy_linux/ToRos/Subsystem ==
  Control : Inport
  Input : Inport  Port=2
  Constant2 : Constant  Value=ampliFactorMiddle  OutDataTypeStr=single
  Dead Zone : DeadZone  LowerValue=0  UpperValue=0.9  SaturateOnIntegerOverflow=on
  Product : Product
  Sum : Sum  Inputs=|++
  "Output " : Outport
  wires:
  Dead Zone/1 -> Sum/1
  Sum/1 -> Product/1
  Constant2/1 -> Sum/2
  Input/1 -> Product/2
  Control/1 -> Dead Zone/1
  Product/1 -> "Output "/1

== system proxy_linux/ToRos/Subsystem1 ==
  Input : Inport
  Constant2 : Constant  Value=ampliFactorDistal  OutDataTypeStr=single
  Dead Zone : DeadZone  LowerValue=0  UpperValue=0.85  SaturateOnIntegerOverflow=on
  Gain : Gain  Gain=1.8  OutDataTypeStr=single
  Product : Product
  Sum : Sum  Inputs=|++
  Output : Outport
  wires:
  Dead Zone/1 -> Gain/1
  Input/1 -> Dead Zone/1, Product/2
  Product/1 -> Output/1
  Constant2/1 -> Sum/2
  Sum/1 -> Product/1
  Gain/1 -> Sum/1

== system proxy_linux/ToRos/Subsystem2 ==
  Control : Inport
  Input : Inport  Port=2
  Constant2 : Constant  Value=ampliFactorMiddle  OutDataTypeStr=single
  Dead Zone : DeadZone  LowerValue=0  UpperValue=0.9  SaturateOnIntegerOverflow=on
  Product : Product
  Sum : Sum  Inputs=|++
  "Output " : Outport
  wires:
  Dead Zone/1 -> Sum/1
  Sum/1 -> Product/1
  Constant2/1 -> Sum/2
  Input/1 -> Product/2
  Control/1 -> Dead Zone/1
  Product/1 -> "Output "/1

== system proxy_linux/ToRos/Subsystem3 ==
  Input : Inport
  Constant2 : Constant  Value=ampliFactorDistal  OutDataTypeStr=single
  Dead Zone : DeadZone  LowerValue=0  UpperValue=0.8  SaturateOnIntegerOverflow=on
  Gain : Gain  Gain=5  OutDataTypeStr=single
  Product : Product
  Sum : Sum  Inputs=|++
  Output : Outport
  wires:
  Dead Zone/1 -> Gain/1
  Input/1 -> Dead Zone/1, Product/2
  Product/1 -> Output/1
  Constant2/1 -> Sum/2
  Sum/1 -> Product/1
  Gain/1 -> Sum/1

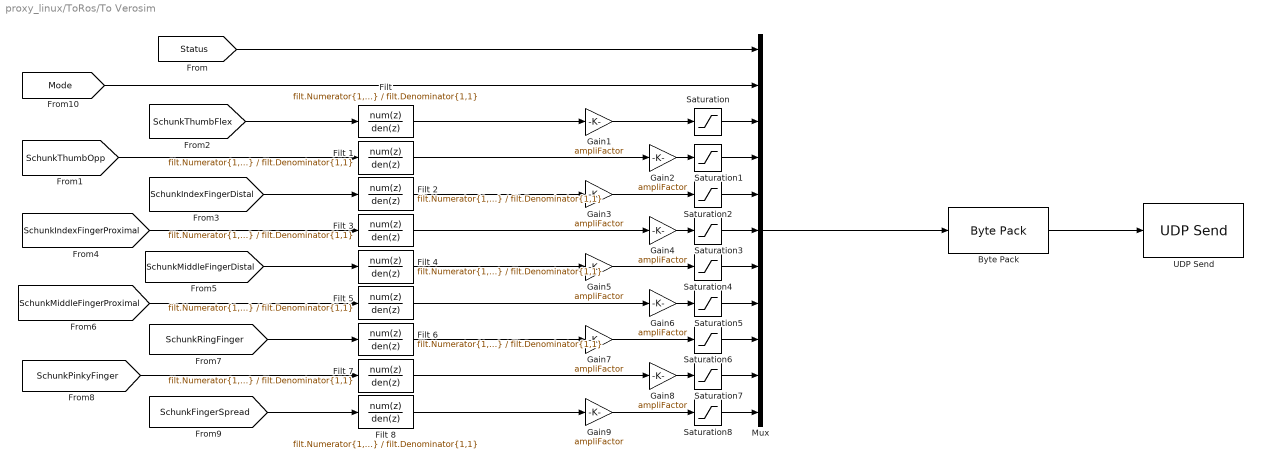
== system proxy_linux/ToRos/To Verosim ==
  Byte Pack : etargetslib/Byte Pack  datatypes={'single'}  byteAlign=1
  Filt {,1..8} (9 alike) : DiscreteTransferFcn  Numerator=filt.Numerator{1,1}  Denominator=filt.Denominator{1,1}  SampleTime=0.01
  Gain{1..9} (9 alike) : Gain  Gain=ampliFactor
  Mux : Mux  Inputs=11
  Saturation : Saturate  UpperLimit=0.97  LowerLimit=0
  Saturation1 : Saturate  UpperLimit=0.99  LowerLimit=0
  Saturation2 : Saturate  UpperLimit=1.33  LowerLimit=0
  Saturation3 : Saturate  UpperLimit=0.80  LowerLimit=0
  Saturation4 : Saturate  UpperLimit=1.33  LowerLimit=0
  Saturation5 : Saturate  UpperLimit=0.80  LowerLimit=0
  Saturation6 : Saturate  UpperLimit=0.98  LowerLimit=0
  Saturation7 : Saturate  UpperLimit=0.98  LowerLimit=0
  Saturation8 : Saturate  UpperLimit=0.58  LowerLimit=0
  UDP Send : dspnetwork/UDP Send  remoteURL='10.100.39.22'  remotePort=15000  localURL='0.0.0.0'  localPortSource=Automatically determine  localPort=-1  sampletime=-1  blockPlatform=HOST  separateLengthPort=0
      settings: SourceProductName=DSP System Toolbox  SourceProductBaseCode=DS
  wires:
  Byte Pack/1 -> UDP Send/1
  Mux/1 -> Byte Pack/1
  [SchunkThumbFlex] -> "Filt "/1
  [SchunkThumbOpp] -> Filt 1/1
  [SchunkIndexFingerDistal] -> Filt 2/1
  [SchunkIndexFingerProximal] -> Filt 3/1
  [SchunkMiddleFingerDistal] -> Filt 4/1
  [SchunkMiddleFingerProximal] -> Filt 5/1
  [SchunkRingFinger] -> Filt 6/1
  [SchunkPinkyFinger] -> Filt 7/1
  [SchunkFingerSpread] -> Filt 8/1
  [Mode] -> Mux/2
  [Status] -> Mux/1
  "Filt "/1 -> Gain1/1
  Filt 1/1 -> Gain2/1
  Filt 2/1 -> Gain3/1
  Filt 3/1 -> Gain4/1
  Filt 4/1 -> Gain5/1
  Filt 5/1 -> Gain6/1
  Filt 6/1 -> Gain7/1
  Filt 7/1 -> Gain8/1
  Filt 8/1 -> Gain9/1
  Gain1/1 -> Saturation/1
  Gain2/1 -> Saturation1/1
  Gain3/1 -> Saturation2/1
  Gain4/1 -> Saturation3/1
  Gain5/1 -> Saturation4/1
  Gain6/1 -> Saturation5/1
  Gain7/1 -> Saturation6/1
  Gain8/1 -> Saturation7/1
  Gain9/1 -> Saturation8/1
  Saturation/1 -> Mux/3
  Saturation1/1 -> Mux/4
  Saturation2/1 -> Mux/5
  Saturation3/1 -> Mux/6
  Saturation4/1 -> Mux/7
  Saturation5/1 -> Mux/8
  Saturation6/1 -> Mux/9
  Saturation7/1 -> Mux/10
  Saturation8/1 -> Mux/11

== system proxy_linux/ToRos/zzz3 ==

== system proxy_linux/Generate SchunkCommands /Finger Spread/calibration1 ==
  In1 : Inport
  Subsystem1 : Subsystem
  Out1 : Outport
  wires:
  [CalibrationSignal] -> Subsystem1/Enable
  In1/1 -> Subsystem1/1(In1)
  Subsystem1/1(Out1) -> Out1/1

== system proxy_linux/Generate SchunkCommands /Index/Calibration ==
  In1 : Inport
  Constant1 : Constant  Value=0.65  OutDataTypeStr=single
  Constant3 : Constant  Value=0.65  OutDataTypeStr=single
  Gain Aggiustato : Gain  Gain=50/1000
  Subsystem : Subsystem
  Sum : Sum  Inputs=|+-
  Sum2 : Sum  Inputs=|++
  Switch : Switch  Criteria=u2 > Threshold
  Out1 : Outport
  wires:
  In1/1 -> Gain Aggiustato/1
  [CalibrationSignal] -> Subsystem/Enable
  Sum/1 -> Sum2/2, Out1/1
  Subsystem/1(Out1) -> Switch/3
  [CalibrationSignal] -> Switch/2
  Constant1/1 -> Switch/1
  Switch/1 -> Sum/2
  Gain Aggiustato/1 -> Sum/1
  Constant3/1 -> Sum2/1
  Sum2/1 -> Subsystem/1(In1)

== system proxy_linux/Generate SchunkCommands /Index/Finger Index  ==
  Mux1 : Mux  Inputs=2
  finger width : Constant  Value=7
  proximal length : Constant  Value=50
  measure : Outport
  wires:
  Mux1/1 -> measure/1
  finger width/1 -> Mux1/1
  proximal length/1 -> Mux1/2

== system proxy_linux/Generate SchunkCommands /Index/Subsystem ==
  Idx Rot : Inport
  Constant : Constant  Value="2*pi  - pi/4 -0.7"  OutDataTypeStr=single
  Constant1 : Constant  Value=-0.185  OutDataTypeStr=single
  Constant2 : Constant  Value=2.34+0.185  OutDataTypeStr=single
  Gain Vero : Gain  Commented=through  Gain=330/1024
  Gain Aggiustato : Gain  Gain=350*pi/(1024*180)
  Radians to Degrees : simulink_extras/Transformations/Radians to Degrees
  Subsystem : Subsystem
  Sum : Sum  Inputs=|+-
  Sum1 : Sum  Inputs=|-+
  Sum2 : Sum  Inputs=|+-
  Switch : Switch  Criteria=u2 > Threshold
  Deg : Outport
  Rad : Outport  Port=2
  tag scope: Index_Precalibration=global
  wires:
  Idx Rot/1 -> Gain Vero/1
  Radians to Degrees/1 -> Deg/1
  Gain Vero/1 -> Gain Aggiustato/1
  Gain Aggiustato/1 -> Sum1/1
  Sum1/1 -> Radians to Degrees/1, Sum2/1, Rad/1
  [CalibrationSignal] -> Switch/2
  Constant/1 -> Sum/1
  Sum/1 -> Sum1/2
  Switch/1 -> Sum/2
  Constant1/1 -> Switch/1
  Constant2/1 -> Sum2/2
  Sum2/1 -> Subsystem/1(In1), [Index_Precalibration]
  [CalibrationSignal] -> Subsystem/Enable
  Subsystem/1(Out1) -> Switch/3

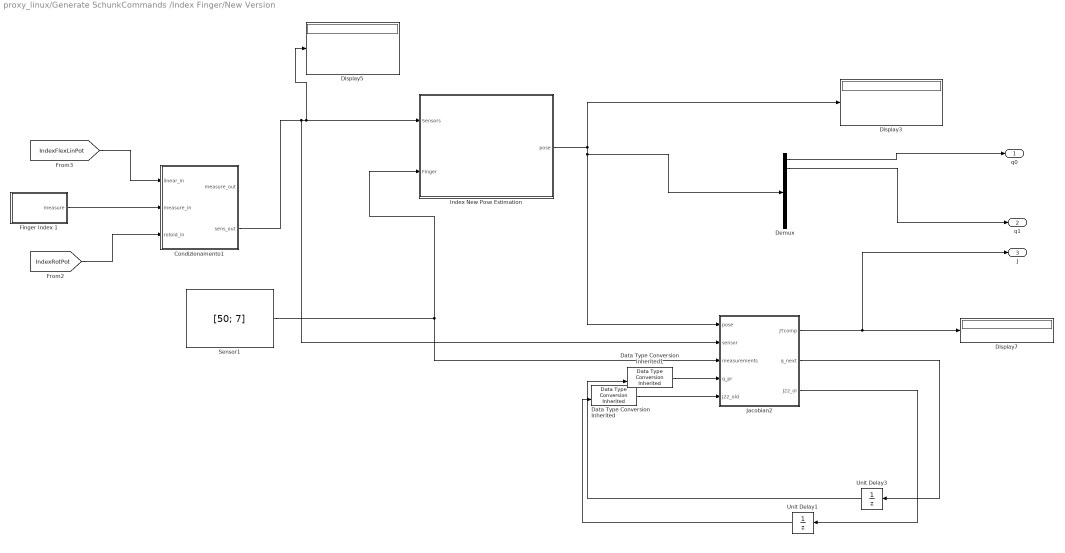
== system proxy_linux/Generate SchunkCommands /Index Finger/New Version ==
  Condizionamento1 : Subsystem
  Data Type Conversion Inherited : simulink/Signal Attributes/Data Type Conversion Inherited  ConvertRealWorld=Real World Value  DoSatur=off
      settings: SourceProductName=Simulink  SourceProductBaseCode=SL
  Data Type Conversion Inherited1 : simulink/Signal Attributes/Data Type Conversion Inherited  ConvertRealWorld=Real World Value  DoSatur=off
      settings: SourceProductName=Simulink  SourceProductBaseCode=SL
  Demux : Demux  Outputs=8
  Display3 : Display
  Display5 : Display
  Display7 : Display
  Finger Index 1 : Subsystem
  "Index New Pose Estimation " : MATLAB Function  TreatAsAtomicUnit=on
  Jacobian2 : MATLAB Function  TreatAsAtomicUnit=on  SystemSampleTime=0.01
  Sensor1 : Constant  Value=[50; 7]
  Unit Delay1 : UnitDelay  InitialCondition=-1  SampleTime=0.01
  Unit Delay3 : UnitDelay  InitialCondition=[0;2.3]  SampleTime=0.01
  q0 : Outport
  q1 : Outport  Port=2
  J : Outport  Port=3
  wires:
  Unit Delay3/1 -> Data Type Conversion Inherited1/2
  Sensor1/1 -> Jacobian2/3(measurements), "Index New Pose Estimation "/2(Finger)
  Data Type Conversion Inherited1/1 -> Jacobian2/4(q_pr)
  Jacobian2/2(q_next) -> Unit Delay3/1
  [IndexRotPot] -> Condizionamento1/3(rotoid_in)
  Finger Index 1/1(measure) -> Condizionamento1/2(measure_in)
  [IndexFlexLinPot] -> Condizionamento1/1(linear_in)
  "Index New Pose Estimation "/1(pose) -> Demux/1, Jacobian2/1(pose), Display3/1
  Unit Delay1/1 -> Data Type Conversion Inherited/2
  Jacobian2/3(J22_ol) -> Unit Delay1/1
  Condizionamento1/2(sens_out) -> Jacobian2/2(sensor), Display5/1, "Index New Pose Estimation "/1(Sensors)
  Data Type Conversion Inherited/1 -> Jacobian2/5(J22_old)
  Jacobian2/1(JTcomp) -> J/1, Display7/1
  Demux/1 -> q0/1
  Demux/2 -> q1/1

== system proxy_linux/Generate SchunkCommands /Index Finger/Old Version ==
  Condizionamento : Subsystem
  Constant : Constant  Value=500  OutDataTypeStr=single
  Constant1 : Constant  Value=0  OutDataTypeStr=single
  "Finger Index " : Subsystem
  MATLAB Function : MATLAB Function  TreatAsAtomicUnit=on
  Manual Switch : ManualSwitch
  Manual Switch1 : ManualSwitch
  Pose Generator : Subsystem
  q0 : Outport
  q1 : Outport  Port=2
  Jacobian : Outport  Port=3
  wires:
  Constant/1 -> MATLAB Function/3(j_f2), MATLAB Function/2(j_f1)
  Pose Generator/2(q_1) -> Manual Switch1/1
  Manual Switch1/1 -> q1/1
  Constant1/1 -> Manual Switch1/2, Manual Switch/2
  Manual Switch/1 -> q0/1
  Pose Generator/1(q_0) -> Manual Switch/1
  Pose Generator/3(J) -> Jacobian/1, MATLAB Function/1(Jcomponents)
  Condizionamento/1(measure_out) -> Pose Generator/2(measures)
  [IndexRotPot] -> Condizionamento/3(rotoid_in)
  Condizionamento/2(sens_out) -> Pose Generator/1("Sensor ")
  "Finger Index "/1(measure) -> Condizionamento/2(measure_in)
  [IndexFlexLinPot] -> Condizionamento/1(linear_in)

== system proxy_linux/Generate SchunkCommands /Middle Finger/Calibration ==
  In1 : Inport
  Constant1 : Constant  Value=11.4  OutDataTypeStr=single
  Constant3 : Constant  Value=11.4  OutDataTypeStr=single
  Gain Aggiustato : Gain  Gain=50/1024
  Subsystem : Subsystem
  Sum : Sum  Inputs=|+-
  Sum2 : Sum  Inputs=|++
  Switch : Switch  Criteria=u2 > Threshold
  Out1 : Outport
  wires:
  In1/1 -> Gain Aggiustato/1
  [CalibrationSignal] -> Switch/2
  Constant1/1 -> Switch/1
  Gain Aggiustato/1 -> Sum/1
  Sum/1 -> Sum2/2, Out1/1
  Switch/1 -> Sum/2
  [CalibrationSignal] -> Subsystem/Enable
  Subsystem/1(Out1) -> Switch/3
  Constant3/1 -> Sum2/1
  Sum2/1 -> Subsystem/1(In1)

== system proxy_linux/Generate SchunkCommands /Middle Finger/Calibration1 ==
  In1 : Inport
  Constant1 : Constant  Value=0  OutDataTypeStr=single
  Constant3 : Constant  Value=0  OutDataTypeStr=single
  Gain Aggiustato : Gain  Gain=50/1024
  Subsystem : Subsystem
  Sum : Sum  Inputs=|+-
  Sum2 : Sum  Inputs=|++
  Switch : Switch  Criteria=u2 > Threshold
  Out1 : Outport
  wires:
  In1/1 -> Gain Aggiustato/1
  [CalibrationSignal] -> Switch/2
  Constant1/1 -> Switch/1
  Gain Aggiustato/1 -> Sum/1
  Sum/1 -> Sum2/2, Out1/1
  Switch/1 -> Sum/2
  [CalibrationSignal] -> Subsystem/Enable
  Subsystem/1(Out1) -> Switch/3
  Constant3/1 -> Sum2/1
  Sum2/1 -> Subsystem/1(In1)

== system proxy_linux/Generate SchunkCommands /Middle Finger/Finger Index  ==
  Mux1 : Mux  Inputs=2
  finger width : Constant  Value=7
  proximal length : Constant  Value=50
  measure : Outport
  wires:
  Mux1/1 -> measure/1
  finger width/1 -> Mux1/1
  proximal length/1 -> Mux1/2

== system proxy_linux/Generate SchunkCommands /Middle Finger/Record ==
  input : Inport
  param : Inport  Port=2
  output : Inport  Port=3
  Enable : EnablePort
  Mux2 : Mux  Inputs=3
  To Workspace : ToWorkspace  VariableName=middle_pose  SampleTime=-1
  wires:
  Mux2/1 -> To Workspace/1
  param/1 -> Mux2/2
  input/1 -> Mux2/1
  output/1 -> Mux2/3

== system proxy_linux/Generate SchunkCommands /Middle Finger/Subsystem ==
  Idx Rot : Inport
  Constant : Constant  Value="2*pi  - pi/4"  OutDataTypeStr=single
  Constant1 : Constant  Value=0.133  OutDataTypeStr=single
  Constant2 : Constant  Value=2.34-0.133  OutDataTypeStr=single
  Gain Vero : Gain  Commented=through  Gain=330/1024
  Gain Aggiustato : Gain  Gain=350*pi/(1024*180)
  Radians to Degrees : simulink_extras/Transformations/Radians to Degrees
  Subsystem : Subsystem
  Sum : Sum  Inputs=|+-
  Sum1 : Sum  Inputs=|-+
  Sum2 : Sum  Inputs=|-+
  Switch : Switch  Criteria=u2 > Threshold
  Deg : Outport
  Rad : Outport  Port=2
  wires:
  Idx Rot/1 -> Gain Vero/1
  Radians to Degrees/1 -> Deg/1
  Gain Vero/1 -> Gain Aggiustato/1
  Gain Aggiustato/1 -> Sum1/1
  Switch/1 -> Sum/2
  [CalibrationSignal] -> Switch/2
  Sum1/1 -> Radians to Degrees/1, Sum2/2, Rad/1
  Constant/1 -> Sum/1
  Sum/1 -> Sum1/2
  Constant2/1 -> Sum2/1
  Constant1/1 -> Switch/1
  Sum2/1 -> Subsystem/1(In1)
  [CalibrationSignal] -> Subsystem/Enable
  Subsystem/1(Out1) -> Switch/3

== system proxy_linux/Generate SchunkCommands /Middle Finger/Subsystem1 ==
  Idx Rot : Inport
  Constant : Constant  Value=3.4+pi/2  OutDataTypeStr=single
  Constant1 : Constant  Value=0  OutDataTypeStr=single
  Constant2 : Constant  Value=3.4+pi/2  OutDataTypeStr=single
  Display : Display
  Display1 : Display
  Gain Vero : Gain  Commented=through  Gain=330/1024
  Gain Aggiustato : Gain  Gain=350*pi/(1024*180)
  Radians to Degrees : simulink_extras/Transformations/Radians to Degrees
  Subsystem : Subsystem
  Sum : Sum  Inputs=|+-
  Sum1 : Sum  Inputs=|-+
  Sum2 : Sum  Inputs=|-+
  Switch : Switch  Criteria=u2 > Threshold
  Deg : Outport
  Rad : Outport  Port=2
  wires:
  Idx Rot/1 -> Gain Vero/1
  Radians to Degrees/1 -> Display1/1, Deg/1
  Gain Vero/1 -> Gain Aggiustato/1
  Gain Aggiustato/1 -> Display/1, Sum1/1
  Switch/1 -> Sum/2
  [CalibrationSignal] -> Switch/2
  Sum1/1 -> Radians to Degrees/1, Sum2/2, Rad/1
  Constant/1 -> Sum/1
  Sum/1 -> Sum1/2
  Constant2/1 -> Sum2/1
  Constant1/1 -> Switch/1
  Sum2/1 -> Subsystem/1(In1)
  [CalibrationSignal] -> Subsystem/Enable
  Subsystem/1(Out1) -> Switch/3

== system proxy_linux/Generate SchunkCommands /Middle Finger/Subsystem2 ==
  In1 : Inport
  In2 : Inport  Port=2
  In3 : Inport  Port=3
  In4 : Inport  Port=4
  Display{1..2,13..14} (4 alike) : Display
  Radians to Degrees{1..4} (4 alike) : simulink_extras/Transformations/Radians to Degrees
  wires:
  Radians to Degrees3/1 -> Display14/1
  In2/1 -> Radians to Degrees3/1
  Radians to Degrees2/1 -> Display13/1
  In1/1 -> Radians to Degrees2/1
  In4/1 -> Radians to Degrees4/1
  Radians to Degrees4/1 -> Display2/1
  Radians to Degrees1/1 -> Display1/1
  In3/1 -> Radians to Degrees1/1

== system proxy_linux/Generate SchunkCommands /Pinky/Subsystem ==
  In1 : Inport
  Enable : EnablePort
  Memory : Memory
  Out1 : Outport
  wires:
  Memory/1 -> Out1/1
  In1/1 -> Memory/1

== system proxy_linux/Generate SchunkCommands /Ring /calibration ==
  In1 : Inport
  Constant2 : Constant  Value=102  OutDataTypeStr=single
  Constant3 : Constant  Value=102  OutDataTypeStr=single
  Display4 : Display
  Subsystem : Subsystem
  Sum2 : Sum  Inputs=|++
  Switch : Switch  Criteria=u2 > Threshold
  Out1 : Outport
  wires:
  [CalibrationSignal] -> Switch/2
  Subsystem/1(Out1) -> Switch/3
  Constant3/1 -> Sum2/1
  [CalibrationSignal] -> Subsystem/Enable
  Constant2/1 -> Switch/1
  Sum2/1 -> Display4/1, Subsystem/1(In1)
  In1/1 -> Sum2/2
  Switch/1 -> Out1/1

== system proxy_linux/Generate SchunkCommands /Thumb/calibration ==
  In1 : Inport
  Constant2 : Constant  Value=540  OutDataTypeStr=single
  Constant3 : Constant  Value=540  OutDataTypeStr=single
  Display4 : Display
  Subsystem : Subsystem
  Sum2 : Sum  Inputs=|++
  Switch : Switch  Criteria=u2 > Threshold
  Out1 : Outport
  wires:
  [CalibrationSignal] -> Switch/2
  Subsystem/1(Out1) -> Switch/3
  Constant3/1 -> Sum2/1
  [CalibrationSignal] -> Subsystem/Enable
  Constant2/1 -> Switch/1
  Sum2/1 -> Display4/1, Subsystem/1(In1)
  In1/1 -> Sum2/2
  Switch/1 -> Out1/1

== system proxy_linux/Generate SchunkCommands /Thumb/calibration1 ==
  In1 : Inport
  Subsystem1 : Subsystem
  Out1 : Outport
  wires:
  [CalibrationSignal] -> Subsystem1/Enable
  In1/1 -> Subsystem1/1(In1)
  Subsystem1/1(Out1) -> Out1/1

== system proxy_linux/Generate SchunkCommands /Finger Spread/calibration1/Subsystem1 ==
  In1 : Inport
  Enable : EnablePort
  Memory : Memory  InitialCondition=460
  Out1 : Outport
  wires:
  Memory/1 -> Out1/1
  In1/1 -> Memory/1

== system proxy_linux/Generate SchunkCommands /Index/Calibration/Subsystem ==
  In1 : Inport
  Enable : EnablePort
  Memory : Memory
  Out1 : Outport
  wires:
  Memory/1 -> Out1/1
  In1/1 -> Memory/1

== system proxy_linux/Generate SchunkCommands /Index/Subsystem/Subsystem ==
  In1 : Inport
  Enable : EnablePort
  Memory : Memory
  Out1 : Outport
  wires:
  Memory/1 -> Out1/1
  In1/1 -> Memory/1

== system proxy_linux/Generate SchunkCommands /Index Finger/New Version/Condizionamento1 ==
  linear_in : Inport
  measure_in : Inport  Port=2
  rotoid_in : Inport  Port=3
  Data Type Conversion : DataTypeConversion  OutDataTypeStr=single
  Display : Display
  Display1 : Display
  Gain Aggiustato : Gain  Gain=50/1000
  Mux : Mux  Inputs=2
  Subsystem : Subsystem
  measure_out : Outport
  sens_out : Outport  Port=2
  wires:
  linear_in/1 -> Gain Aggiustato/1
  Subsystem/1(Deg) -> Display/1
  Gain Aggiustato/1 -> Mux/1
  Data Type Conversion/1 -> measure_out/1
  measure_in/1 -> Data Type Conversion/1
  Subsystem/2(Rad) -> Mux/2, Display1/1
  rotoid_in/1 -> Subsystem/1(Idx Rot)
  Mux/1 -> sens_out/1

== system proxy_linux/Generate SchunkCommands /Index Finger/New Version/Finger Index 1 ==
  Mux1 : Mux  Inputs=2
  finger width : Constant  Value=10
  proximal length : Constant  Value=50
  measure : Outport
  wires:
  Mux1/1 -> measure/1
  finger width/1 -> Mux1/1
  proximal length/1 -> Mux1/2
